simulink model "DO_rnd_shift"  (R2023b)
settings: Solver=VariableStepAuto  StartTime=0.0  StopTime=inf  RelTol=1e-3
values from neighbouring files (symbols this model uses):
  bit_sample_index = i    [eval_agent.m]
  bit_seq = zeros(1,sample_length)    [eval_agent.m]
  diff_training_n = bit_seq_split.*repeated_values    [eval_agent.m]
  initial_n = -1    [eval_agent.m]
  is_training = false    [eval_agent.m]
  max_initial_n = 1    [eval_agent.m]
  mol_seq = mol_seq(1 : sample_step : length(mol_seq))    [eval_agent.m]
  mols_action_max = 100    [eval_agent.m]
  mols_action_min = -100    [eval_agent.m]
  mols_action_step = 10    [eval_agent.m]
  mols_max = 360    [eval_agent.m]
  mols_min = 0    [eval_agent.m]
  obs_max = 200    [eval_agent.m]
  obs_min = -200    [eval_agent.m]
  obs_step = 5    [eval_agent.m]
  sample_length = length(sec_axis)    [eval_agent.m]
  snr = 30    [eval_agent.m]
  stop_time = transmissions_per_interval * num_intervals    (= 5000)    [eval_agent.m]
  switch_index = false    [eval_agent.m]
  use_training_reward = false    [eval_agent.m]
libraries: simulink x2, commrandsrc3 x2, rllib x1
settings Model: Creator=black  LastModifiedBy=lyd

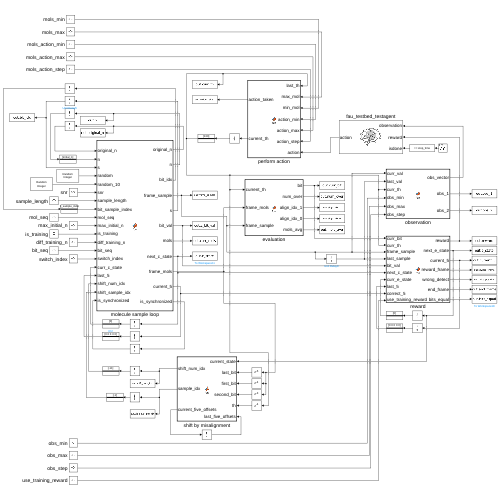
[thumbnail: Simulink's stored preview of the top-level diagram]
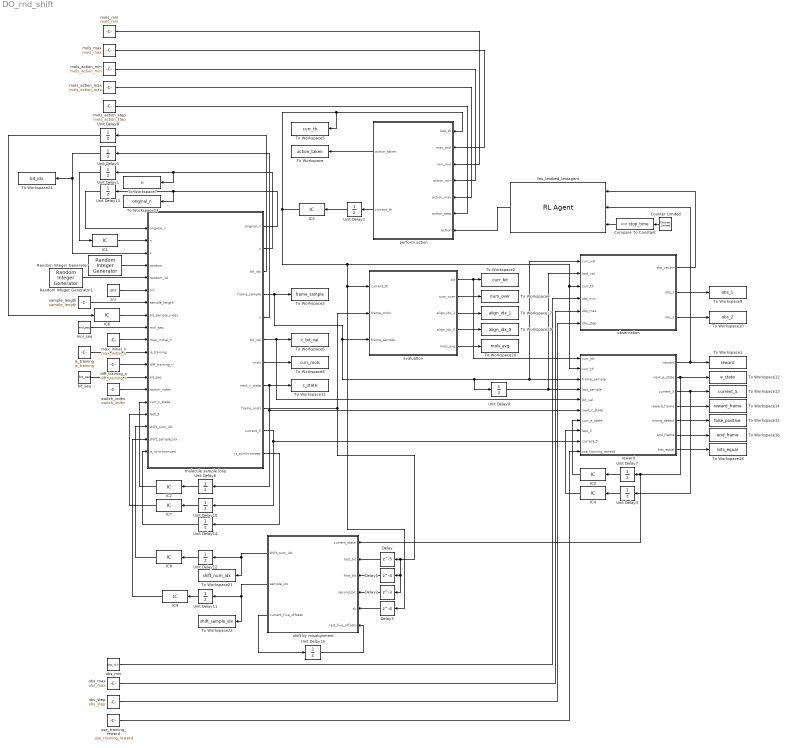
== system DO_rnd_shift ==
  Compare To Constant : simulink/Logic and Bit Operations/Compare To Constant  relop===  const=stop_time  OutDataTypeStr=boolean
  Counter Limited : simulink/Sources/Counter Limited  uplimit=stop_time  tsamp=1
  Delay : Delay  DelayLength=5  InitialCondition=0
  Delay1 : Delay  DelayLength=4  InitialCondition=0
  Delay2 : Delay  DelayLength=3  InitialCondition=0
  Delay3 : Delay  DelayLength=4  InitialCondition=0
  IC1 : InitialCondition  Value=initial_n
  IC2 : InitialCondition  Value=0
  IC3 : InitialCondition  Value=0
  IC4 : InitialCondition  Value=[0 0 0 0 0]
  IC5 : InitialCondition  Value=130
  IC6 : InitialCondition  Value=bit_sample_index
  IC7 : InitialCondition  Value=[0 0 0 0 0]
  IC8 : InitialCondition  Value=-11
  IC9 : InitialCondition  Value=-1
  Random Integer Generator : commrandsrc3/Random Integer Generator  SetSize=8  SeedSource=Auto  Seed=0  SampleTime=1  SamplesPerFrame=1  OutputDataType=double  SimulateUsing=Interpreted execution
  Random Integer Generator1 : commrandsrc3/Random Integer Generator  SetSize=9  SeedSource=Auto  Seed=0  SampleTime=1  SamplesPerFrame=1  OutputDataType=double  SimulateUsing=Interpreted execution
  To Workspace : ToWorkspace  VariableName=action_taken  SaveFormat=Timeseries  SampleTime=-1
  To Workspace1 : ToWorkspace  VariableName=reward  SaveFormat=Timeseries  SampleTime=-1
  To Workspace10 : ToWorkspace  VariableName=obs_2  SaveFormat=Timeseries  SampleTime=-1
  To Workspace11 : ToWorkspace  VariableName=c_state  SaveFormat=Timeseries  SampleTime=-1
  To Workspace12 : ToWorkspace  VariableName=e_state  SaveFormat=Timeseries  SampleTime=-1
  To Workspace13 : ToWorkspace  VariableName=current_5  SaveFormat=Timeseries  SampleTime=-1
  To Workspace14 : ToWorkspace  VariableName=reward_frame  SaveFormat=Timeseries  SampleTime=-1
  To Workspace15 : ToWorkspace  VariableName=false_positive  SaveFormat=Timeseries  SampleTime=-1
  To Workspace16 : ToWorkspace  VariableName=end_frame  SaveFormat=Timeseries  SampleTime=-1
  To Workspace17 : ToWorkspace  VariableName=align_idx_1  SaveFormat=Timeseries  SampleTime=-1
  To Workspace18 : ToWorkspace  VariableName=bits_equal  SaveFormat=Timeseries  SampleTime=-1
  To Workspace19 : ToWorkspace  VariableName=align_idx_0  SaveFormat=Timeseries  SampleTime=-1
  To Workspace2 : ToWorkspace  VariableName=curr_bit  SaveFormat=Timeseries  SampleTime=-1
  To Workspace20 : ToWorkspace  VariableName=mols_avg  SaveFormat=Timeseries  SampleTime=-1
  To Workspace21 : ToWorkspace  VariableName=shift_num_idx  SaveFormat=Timeseries  SampleTime=-1
  To Workspace22 : ToWorkspace  VariableName=shift_sample_idx  SaveFormat=Timeseries  SampleTime=-1
  To Workspace23 : ToWorkspace  VariableName=original_n  SaveFormat=Timeseries  SampleTime=-1
  To Workspace24 : ToWorkspace  VariableName=bit_idx  SaveFormat=Timeseries  SampleTime=-1
  To Workspace3 : ToWorkspace  VariableName=frame_sample  SaveFormat=Timeseries  SampleTime=-1
  To Workspace4 : ToWorkspace  VariableName=num_over  SaveFormat=Timeseries  SampleTime=-1
  To Workspace5 : ToWorkspace  VariableName=curr_th  SaveFormat=Timeseries  SampleTime=-1
  To Workspace6 : ToWorkspace  VariableName=c_bit_val  SaveFormat=Timeseries  SampleTime=-1
  To Workspace7 : ToWorkspace  VariableName=n  SaveFormat=Timeseries  SampleTime=-1
  To Workspace8 : ToWorkspace  VariableName=curr_mols  SaveFormat=Timeseries  SampleTime=-1
  To Workspace9 : ToWorkspace  VariableName=obs_1  SaveFormat=Timeseries  SampleTime=-1
  Unit Delay{1..3,5..15} (14 alike) : UnitDelay  SampleTime=-1  HasFrameUpgradeWarning=on
  bit_seq : Constant  Value=bit_seq  SampleTime=1
  diff_training_n : Constant  Value=diff_training_n  SampleTime=1
  evaluation : MATLAB Function  TreatAsAtomicUnit=on
  fau_testbed_testagent : rllib/RL Agent  Agent=agent  ExternalActionAsInput=off  ProvideLastAction=off  ProvideCumRwd=off  TreatAsDirectFeedthrough=on  UseStrictObservationDataTypes=off
  is_training : Constant  Value=is_training  SampleTime=1
  max_initial_n : Constant  Value=max_initial_n  SampleTime=1
  mol_seq : Constant  Value=mol_seq  SampleTime=1
  molecule sample loop : MATLAB Function  TreatAsAtomicUnit=on
  mols_action_max : Constant  Value=mols_action_max  SampleTime=1
  mols_action_min : Constant  Value=mols_action_min  SampleTime=1
  mols_action_step : Constant  Value=mols_action_step  SampleTime=1
  mols_max : Constant  Value=mols_max  SampleTime=1
  mols_min : Constant  Value=mols_min  SampleTime=1
  obs_max : Constant  Value=obs_max  SampleTime=1
  obs_min : Constant  Value=obs_min  SampleTime=1
  obs_step : Constant  Value=obs_step  SampleTime=1
  observation : MATLAB Function  TreatAsAtomicUnit=on
  perform action : MATLAB Function  TreatAsAtomicUnit=on
  reward : MATLAB Function  TreatAsAtomicUnit=on
  sample_length : Constant  Value=sample_length  SampleTime=1
  shift by misalignment : MATLAB Function  TreatAsAtomicUnit=on
  snr : Constant  Value=snr  SampleTime=1
  switch_index : Constant  Value=switch_index  SampleTime=1
  use_training_reward : Constant  Value=use_training_reward  SampleTime=1
  wires:
  Unit Delay1/1 -> IC1/1
  molecule sample loop/2(n) -> To Workspace7/1, Unit Delay1/1
  IC1/1 -> molecule sample loop/2("n ")
  mol_seq/1 -> molecule sample loop/9(mol_seq)
  sample_length/1 -> molecule sample loop/7(sample_length)
  Unit Delay2/1 -> IC5/1
  perform action/2(current_th) -> Unit Delay2/1
  fau_testbed_testagent/1 -> perform action/7(action)
  Counter Limited/1 -> Compare To Constant/1
  Compare To Constant/1 -> fau_testbed_testagent/3
  reward/1(reward) -> fau_testbed_testagent/2, To Workspace1/1
  perform action/1(action_taken) -> To Workspace/1
  evaluation/1(bit) -> reward/1(curr_bit), To Workspace2/1
  observation/1(obs_vector) -> fau_testbed_testagent/1
  max_initial_n/1 -> molecule sample loop/10(max_initial_n)
  molecule sample loop/4(frame_sample) -> To Workspace3/1, observation/1(curr_val), reward/3(frame_sample), Unit Delay9/1, evaluation/3(frame_sample)
  molecule sample loop/5(s) -> Unit Delay5/1
  Unit Delay5/1 -> To Workspace24/1, molecule sample loop/3("s ")
  is_training/1 -> molecule sample loop/11(is_training)
  diff_training_n/1 -> molecule sample loop/12(diff_training_n)
  Random Integer Generator/1 -> molecule sample loop/4(random)
  molecule sample loop/6(bit_val) -> reward/5(bit_val), To Workspace6/1
  bit_seq/1 -> molecule sample loop/13(bit_seq)
  molecule sample loop/7(mols) -> To Workspace8/1
  IC6/1 -> molecule sample loop/8(bit_sample_index)
  mols_min/1 -> perform action/3(min_mol)
  mols_max/1 -> perform action/2(max_mol)
  observation/2(obs_1) -> To Workspace9/1
  snr/1 -> molecule sample loop/6(snr)
  molecule sample loop/8(next_c_state) -> Unit Delay6/1, reward/6(next_c_state), To Workspace11/1
  Unit Delay6/1 -> IC2/1
  IC2/1 -> molecule sample loop/15(curr_c_state)
  reward/2(next_e_state) -> To Workspace12/1, shift by misalignment/1(current_state), Unit Delay7/1
  Unit Delay7/1 -> IC3/1
  IC3/1 -> reward/7(curr_e_state)
  mols_action_max/1 -> perform action/5(action_max)
  mols_action_min/1 -> perform action/4(action_min)
  mols_action_step/1 -> perform action/6(action_step)
  molecule sample loop/9(frame_mols) -> evaluation/2(frame_mols), Delay1/1, Delay2/1, Delay/1
  IC5/1 -> To Workspace5/1, perform action/1(last_th), reward/2(curr_th), observation/3(curr_th), Delay3/1, evaluation/1(current_th)
  evaluation/2(num_over) -> To Workspace4/1
  obs_min/1 -> observation/4(obs_min)
  obs_max/1 -> observation/5(obs_max)
  obs_step/1 -> observation/6(obs_step)
  observation/3(obs_2) -> To Workspace10/1
  Unit Delay3/1 -> IC4/1
  IC4/1 -> reward/8(last_5)
  reward/3(current_5) -> To Workspace13/1, Unit Delay3/1
  reward/4(reward_frame) -> To Workspace14/1
  reward/5(wrong_detect) -> To Workspace15/1
  reward/6(end_frame) -> To Workspace16/1
  evaluation/3(align_idx_1) -> To Workspace17/1
  reward/7(bits_equal) -> To Workspace18/1
  evaluation/4(align_idx_0) -> To Workspace19/1
  use_training_reward/1 -> reward/10(use_training_reward)
  evaluation/5(mols_avg) -> To Workspace20/1
  switch_index/1 -> molecule sample loop/14(switch_index)
  molecule sample loop/3(bit_idx) -> Unit Delay8/1
  Unit Delay8/1 -> IC6/1
  Random Integer Generator1/1 -> molecule sample loop/5(random_10)
  Unit Delay9/1 -> observation/2(last_val), reward/4(last_sample)
  IC7/1 -> molecule sample loop/16(last_5)
  molecule sample loop/10(current_5) -> Unit Delay10/1, reward/9(correct_5)
  Unit Delay10/1 -> IC7/1
  Delay/1 -> shift by misalignment/2(last_bit)
  Delay1/1 -> shift by misalignment/3(first_bit)
  Delay2/1 -> shift by misalignment/4(second_bit)
  Delay3/1 -> shift by misalignment/5(th)
  shift by misalignment/1(shift_num_idx) -> To Workspace21/1, Unit Delay12/1
  shift by misalignment/2(sample_idx) -> To Workspace22/1, Unit Delay11/1
  Unit Delay11/1 -> IC9/1
  Unit Delay12/1 -> IC8/1
  IC8/1 -> molecule sample loop/17(shift_num_idx)
  IC9/1 -> molecule sample loop/18(shift_sample_idx)
  molecule sample loop/1(original_n) -> To Workspace23/1, Unit Delay13/1
  Unit Delay13/1 -> molecule sample loop/1("original_n ")
  molecule sample loop/11(is_synchronized) -> Unit Delay14/1
  Unit Delay14/1 -> molecule sample loop/19("is_synchronized ")
  Unit Delay15/1 -> shift by misalignment/6(last_five_offsets)
  shift by misalignment/3(current_five_offsets) -> Unit Delay15/1

== matlab function DO_rnd_shift/evaluation ==
  data: current_th input; frame_mols input size=10; bit output double size=1; frame_sample input; num_over output; align_idx_1 output; align_idx_0 output; mols_avg output
function [bit, num_over, align_idx_1, align_idx_0, mols_avg] = fcn(current_th, frame_mols, frame_sample)

% check for misaliagnment in possible cases
num_over = nnz(frame_mols >= current_th);
idx = find(frame_mols >= current_th, 1 );
align_idx_1 = -1;
if ~isempty(idx)
    align_idx_1 = idx(1);
end
idx = find(frame_mols < current_th, 1 );
align_idx_0 = -1;
if ~isempty(idx)
    align_idx_0 = idx(1);
end

% threshold decoder
bit = 0;
if(frame_sample(1) >= current_th)
    bit = 1;
end

mols_avg = mean(frame_mols);

== matlab function DO_rnd_shift/observation ==
  data: curr_val input double size=3; last_val input; curr_th input; obs_vector output size=[1 2]; obs_1 output; obs_min input; obs_max input; obs_step input; obs_2 output
function [obs_vector, obs_1, obs_2] = fcn(curr_val, last_val, curr_th, obs_min, obs_max, obs_step)

% content of frame sample:
% frame_sample(1) = frame_mols(bit_sample_index);
% frame_sample(2) = max(frame_mols);
% frame_sample(3) = min(frame_mols);
% ONLY USE INDEX 1 IN THE OBSERVATIONS!

% calculate observation values
obs_1 = curr_val(1) - curr_th;
obs_2 = curr_val(1) - last_val(1);

% round observation values according to agent definition
if obs_1 < obs_min
    obs_1 = obs_min;
elseif obs_1 > obs_max
    obs_1 = obs_max;
end
if obs_2 < obs_min
    obs_2 = obs_min;
elseif obs_2 > obs_max
    obs_2 = obs_max;
end
obs_lower = obs_min - obs_step;
obs_upper = obs_max + obs_step;
obs_1 = interp1([obs_lower:obs_step:obs_upper],[obs_lower:obs_step:obs_upper],[obs_1],'nearest');
obs_2 = interp1([obs_lower:obs_step:obs_upper],[obs_lower:obs_step:obs_upper],[obs_2],'nearest');

% set observations
obs_vector = [obs_1 obs_2];

== matlab function DO_rnd_shift/shift by misalignment ==
  data: current_state input; last_bit input size=10; shift_num_idx output double size=1; first_bit input; second_bit input; sample_idx output; th input; last_five_offsets input; current_five_offsets output
function [shift_num_idx, sample_idx, current_five_offsets] = fcn(current_state, last_bit, first_bit, second_bit, th, last_five_offsets)

% prep variables
found_sync = false;
if current_state == 10
    found_sync = true;
end
current_five_offsets = zeros(5,1);
if (current_five_offsets == [00000])
    reset_offsets = true;
end
sample_idx = -1;

% check for misalignment and set sampling offset
if found_sync
    transition = [last_bit(10); first_bit(1:2)];
    indexes = find(transition >= th);
    if ~isempty(indexes)
        shift_num_idx = indexes(1) - 1;
        if shift_num_idx < 0
            shifted_bit = [last_bit(shift_num_idx+11:10); first_bit(1:shift_num_idx+10)];
            [~,sample_idxes] = max(shifted_bit);
        elseif shift_num_idx == 0
            [~,sample_idxes] = max(first_bit);
        else
            shifted_bit = [first_bit(1+shift_num_idx:10); second_bit(1:shift_num_idx)];
            [~,sample_idxes] = max(shifted_bit);
        end
    else
        shift_num_idx = 1;
        shifted_bit = [first_bit(1+shift_num_idx:10); second_bit(1:shift_num_idx)];
        [~,sample_idxes] = max(shifted_bit);
    end

    current_five_offsets(1,1) = last_five_offsets(2,1);
    current_five_offsets(2,1) = last_five_offsets(3,1);
    current_five_offsets(3,1) = last_five_offsets(4,1);
    current_five_offsets(4,1) = last_five_offsets(5,1);
    current_five_offsets(5,1) = sample_idxes(1,1) + shift_num_idx;
    if reset_offsets
        current_five_offsets(1,1) = current_five_offsets(5,1);
        current_five_offsets(2,1) = current_five_offsets(5,1);
        current_five_offsets(3,1) = current_five_offsets(5,1);
        current_five_offsets(4,1) = current_five_offsets(5,1);
    end
    idx = round(mean(current_five_offsets));
    sample_idx = idx(1,1);

    if sample_idx <= 0
        sample_idx = 1;
    end
    if sample_idx > 10
        sample_idx = 10;
    end

else
    current_five_offsets(1,1) = last_five_offsets(1,1);
    current_five_offsets(2,1) = last_five_offsets(2,1);
    current_five_offsets(3,1) = last_five_offsets(3,1);
    current_five_offsets(4,1) = last_five_offsets(4,1);
    current_five_offsets(5,1) = last_five_offsets(5,1);
    shift_num_idx = -11;
    sample_idx = -1;
end

== matlab function DO_rnd_shift/perform action ==
  data: action_taken output double size=1; last_th input size=1; max_mol input size=1; min_mol input size=1; action_min input; action_max input; action_step input; action input double size=1; current_th output double size=1
function [action_taken, current_th]  = fcn(last_th, max_mol, min_mol, action_min, action_max, action_step, action)

% adapt threshold according to action
current_th = last_th + action;
if current_th < min_mol
    current_th = min_mol;
elseif current_th > max_mol
    current_th = max_mol;
end

action_taken = action;

== matlab function DO_rnd_shift/reward ==
  data: reward output double size=1; curr_bit input size=1; curr_th input size=1; frame_sample input; last_sample input; bit_val input size=1; next_c_state input; curr_e_state input; next_e_state output; last_5 input; correct_5 input; current_5 output; reward_frame output; wrong_detect output; end_frame output; bits_equal output; use_training_reward input
function [reward, next_e_state, current_5, reward_frame, wrong_detect, end_frame, bits_equal] = fcn(curr_bit, curr_th, frame_sample, last_sample, bit_val, next_c_state, curr_e_state, last_5, correct_5, use_training_reward)

% prep variables
bit_is_one = curr_bit == 1;
bits_equal = curr_bit == bit_val;
current_5 = zeros(5,1);
current_5(1) = last_5(2);
current_5(2) = last_5(3);
current_5(3) = last_5(4);
current_5(4) = last_5(5);
current_5(5) = curr_bit;

% correlator state machine
switch curr_e_state
    case 0
        if bit_is_one
            next_e_state = 2;
        else
            next_e_state = 11;
        end
    case 2
        if bit_is_one
            next_e_state = 4;
        else
            next_e_state = 14;
        end
    case 4
        if ~bit_is_one
            next_e_state = 6;
        else
            next_e_state = 16;
        end
    case 6
        if ~bit_is_one
            next_e_state = 8;
        else
            next_e_state = 18;
        end
    case 8
        if bit_is_one
            next_e_state = 10;
        else
            next_e_state = 20;
        end
    case 10
        if bit_is_one
            next_e_state = 2;
        else
            next_e_state = 12;
        end
    case 11
        if bit_is_one
            next_e_state = 2;
        else
            next_e_state = 12;
        end
    case 12
        next_e_state = 14;
    case 14
        next_e_state = 16;
    case 16
        next_e_state = 18;
    case 18
        next_e_state = 20;
    case 20
        if bit_is_one
            next_e_state = 2;
        else
            next_e_state = 12;
        end
    otherwise
        error("wrong state "+curr_e_state);
end

% reset for new time-series
if next_c_state == 11
    next_e_state = 11;
end

% output frame state
wrong_detect = false;
end_frame = false;
if next_c_state == 10 || next_c_state == 20
    end_frame = true;
end

% set the value the reward aims for
sample_goal = frame_sample(1);
if last_sample(1) > frame_sample(1)
    sample_goal = (last_sample(1) - frame_sample(1))/2+frame_sample(1);
else
    sample_goal = (frame_sample(1) - last_sample(1))/2+last_sample(1);
end

% constants for reward calculation
max_diff = 0;
max_diff_frame = max_diff * 0;

% calculate reward
if use_training_reward
    reward_frame = 0;
    if (next_c_state == 10 || next_c_state == 20) && isequal(current_5, correct_5)
        reward_frame = max_diff_frame;
    elseif isequal(current_5, [1;1;0;0;1]) && (next_c_state > 10 || next_c_state < -10)
        wrong_detect = true;
    end
    reward_th_diff = abs(sample_goal - curr_th);
    reward_bit_val = 0;
    if (bits_equal)
        reward_bit_val = max_diff;
    end
else
    reward_frame = 0;
    if next_e_state == 10 && isequal(current_5, [1;1;0;0;1])
        reward_frame = max_diff_frame; 
    elseif next_e_state == 20 && ~isequal(current_5, [1;1;0;0;1])
        reward_frame = 0;
    elseif isequal(current_5, [1;1;0;0;1]) && (next_c_state > 10 || next_c_state < -10)
        wrong_detect = true;
    end
    reward_th_diff = abs(sample_goal - curr_th);
    reward_bit_val = 0;
    if (next_e_state >= 0)
        reward_bit_val = max_diff;
    end
end

reward_th_diff = reward_th_diff * reward_th_diff;
reward = reward_bit_val * 1 - reward_th_diff + reward_frame; %a:75, b:30, c:100+^2, d:65
reward = reward / 100;

next_o_state = next_c_state;

== matlab function DO_rnd_shift/molecule sample loop ==
  data: original_n output; original_n input; n input double size=1; s input; random input; random_10 input; snr input; sample_length input double size=1; bit_sample_index input; n output; bit_idx output; mol_seq input; frame_sample output size=3; max_initial_n input size=1; s output; is_training input; diff_training_n input; bit_seq input; switch_index input; bit_val output; mols output; curr_c_state input; next_c_state output; frame_mols output; last_5 input; current_5 output; shift_num_idx input; shift_sample_idx input; is_synchronized input; is_synchronized output
function [original_n, n, bit_idx, frame_sample, s, bit_val, mols, next_c_state,frame_mols, current_5, is_synchronized] = fcn(original_n, n, s, random, random_10, snr, sample_length, bit_sample_index, mol_seq, max_initial_n, is_training, diff_training_n, bit_seq, switch_index, curr_c_state, last_5, shift_num_idx, shift_sample_idx, is_synchronized)

% check current sampling index
bit_idx = bit_sample_index;
if shift_sample_idx > 0
    bit_idx = shift_sample_idx;
    is_synchronized = 1;
end

% set current timerseries
if is_training
    if s == 0
        s = 1;
    end
    if (n+10 > length(mol_seq) || n < 1)
        s = mod(random, length(diff_training_n)) + 1;
        n = max_initial_n + sum(diff_training_n(1:s-1));
        original_n = n;
        curr_c_state = 0;
        is_synchronized = 0;
        if switch_index
            bit_idx = random_10 + 1;
        end
    end
else
    s = -1;
    if n < 1
        n = randi(max_initial_n);
        original_n = n;
        is_synchronized = 0;
        if switch_index
            bit_idx = random_10 + 1;
        end
    end
    if (n+10 > length(mol_seq))
        n = max_initial_n;
        original_n = n;
        is_synchronized = 0;
        if switch_index
            bit_idx = random_10 + 1;
        end
    end
    for i = 1:length(diff_training_n)
        if n == max_initial_n + sum(diff_training_n(1:i-1))
            curr_c_state = 0;
            n = original_n;
            is_synchronized = 0;
        end
    end
end

% sample the next bit
% add wgn
frame_mols = zeros(10,1);
frame_mols_complete = zeros(20,1);
if n - 10 > 0
    frame_mols_complete(1:20) = awgn(mol_seq(n - 10 : (10 + n - 1)), snr, 'measured');
else
    frame_mols_complete(11:20) = awgn(mol_seq(n : (10 + n - 1)), snr, 'measured');
end
frame_mols(1:10) = frame_mols_complete(11:20);

% set frame samples 
frame_sample = zeros(3, 1);
frame_sample(1) = frame_mols(bit_idx);
frame_sample(2) = max(frame_mols);
frame_sample(3) = min(frame_mols);

obs_frame_mols = zeros(10,1);
if is_synchronized > 0
    obs_frame_mols = frame_mols_complete(bit_idx + 1: bit_idx + 10);
    frame_sample(2) = mean(obs_frame_mols);
    frame_sample(3) = min(obs_frame_mols);
end

mols = frame_mols(bit_idx);

bit_val = 0;
if (bit_seq(original_n + 1) == 1)
    bit_val = 1;
end

bit_is_one = bit_val == 1;

% pass through state machine for expected states
switch curr_c_state
    case 0
        if bit_is_one
            next_c_state = 2;
        else
            next_c_state = 11;
        end
    case 2
        if bit_is_one
            next_c_state = 4;
        else
            next_c_state = 14;
        end
    case 4
        if ~bit_is_one
            next_c_state = 6;
        else
            next_c_state = 16;
        end
    case 6
        if ~bit_is_one
            next_c_state = 8;
        else
            next_c_state = 18;
        end
    case 8
        if bit_is_one
            next_c_state = 10;
        else
            next_c_state = 20;
        end
    case 10
        if bit_is_one
            next_c_state = 2;
        else
            next_c_state = 12;
        end
    case 11
        if bit_is_one
            next_c_state = 2;
        else
            next_c_state = 12;
        end
    case 12
        next_c_state = 14;
    case 14
        next_c_state = 16;
    case 16
        next_c_state = 18;
    case 18
        next_c_state = 20;
    case 20
        if bit_is_one
            next_c_state = 2;
        else
            next_c_state = 12;
        end
    otherwise
        error("wrong state "+curr_c_state);
end

% increment n
if n + 10 > sample_length
    n = 1;
else
    n = n + 10;
end

if original_n + 10 > sample_length
    original_n = 1;
else
    original_n = original_n + 10;
end


current_5 = zeros(5,1);
current_5(1,1) = last_5(2,1);
current_5(2,1) = last_5(3,1);
current_5(3,1) = last_5(4,1);
current_5(4,1) = last_5(5,1);
current_5(5,1) = bit_is_one;
